simulink model "Clik_Jacobian_second_order"  (R2023a)
settings: Solver=VariableStepAuto  StartTime=0.0  StopTime=20  RelTol=1e-6
model workspace: external: MAT-File (data not in the file)
undefined symbols (not defined in the file): DiscIntNeverNeededParam, f_s
settings Model: Creator=benit  LastModifiedBy=Savio Del Peschio
settings OptimizationCC: ReuseModelBlockBuffer=off

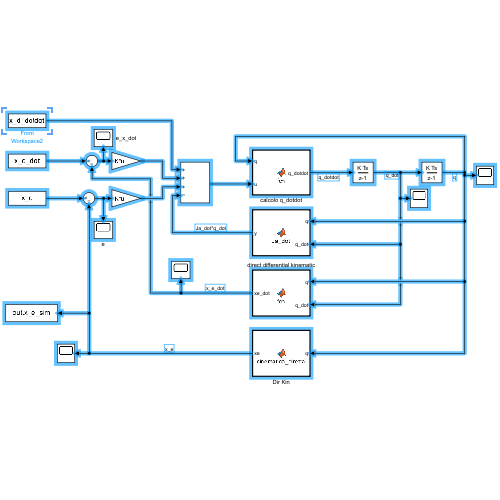
[thumbnail: Simulink's stored preview of the top-level diagram]
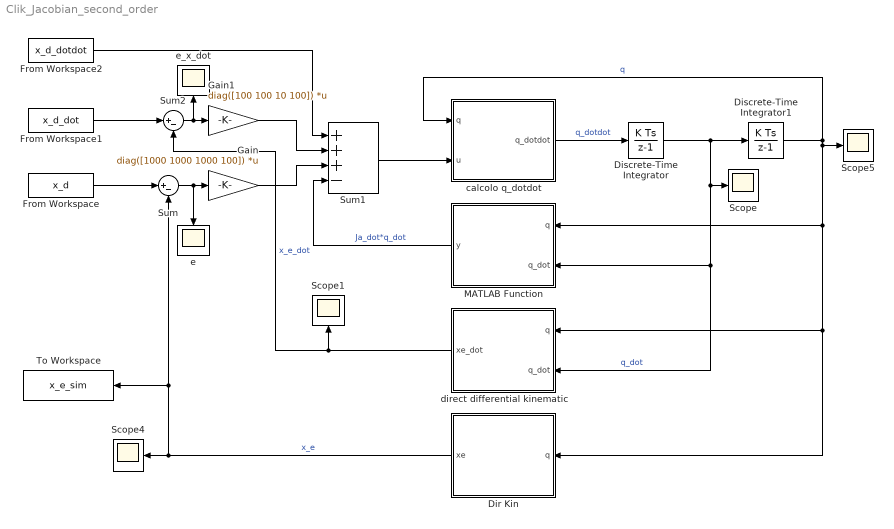
== system Clik_Jacobian_second_order ==
  Dir Kin : MATLAB Function  TreatAsAtomicUnit=on
  Discrete-Time Integrator : DiscreteIntegrator  gainval=1  InitialCondition=zeros(4,1)  SampleTime=1/f_s  ICPrevOutput=DiscIntNeverNeededParam  ICPrevScaledInput=DiscIntNeverNeededParam
  Discrete-Time Integrator1 : DiscreteIntegrator  gainval=1  InitialCondition=config_p_init'  SampleTime=1/f_s  ICPrevOutput=DiscIntNeverNeededParam  ICPrevScaledInput=DiscIntNeverNeededParam
  From Workspace : FromWorkspace  VariableName=x_d
  From Workspace1 : FromWorkspace  VariableName=x_d_dot
  From Workspace2 : FromWorkspace  VariableName=x_d_dotdot
  Gain : Gain  Gain=diag([1000 1000 1000 100])  Multiplication=Matrix(K*u)
  Gain1 : Gain  Gain=diag([100 100 10 100])  Multiplication=Matrix(K*u)
  MATLAB Function : MATLAB Function  TreatAsAtomicUnit=on
  Scope{,1,4..5} (4 alike) : Scope
  Sum : Sum  Inputs=|+-
  Sum1 : Sum  Inputs=+++-
  Sum2 : Sum  Inputs=|+-
  To Workspace : ToWorkspace  VariableName=x_e_sim  SaveFormat=Timeseries  SampleTime=-1
  calcolo q_dotdot : MATLAB Function  TreatAsAtomicUnit=on
  direct differential kinematic : MATLAB Function  TreatAsAtomicUnit=on
  e : Scope
  e_x_dot : Scope
  wires:
  calcolo q_dotdot/1(q_dotdot) -> Discrete-Time Integrator/1  "q_dotdot"
  From Workspace/1 -> Sum/1
  Dir Kin/1(xe) -> To Workspace/1, Sum/2, Scope4/1  "x_e"
  From Workspace1/1 -> Sum2/1
  Sum2/1 -> e_x_dot/1, Gain1/1
  From Workspace2/1 -> Sum1/1
  Gain1/1 -> Sum1/2
  Gain/1 -> Sum1/3
  direct differential kinematic/1(xe_dot) -> Sum2/2, Scope1/1  "x_e_dot"
  Sum1/1 -> calcolo q_dotdot/2(u)
  MATLAB Function/1(y) -> Sum1/4  "Ja_dot*q_dot"
  Discrete-Time Integrator/1 -> direct differential kinematic/2(q_dot), MATLAB Function/2(q_dot), Scope/1, Discrete-Time Integrator1/1  "q_dot"
  Discrete-Time Integrator1/1 -> Scope5/1, Dir Kin/1(q), direct differential kinematic/1(q), MATLAB Function/1(q), calcolo q_dotdot/1(q)  "q"
  Sum/1 -> e/1, Gain/1

== matlab function Clik_Jacobian_second_order/calcolo q_dotdot ==
  data: q input; u input; q_dotdot output
function q_dotdot = fcn(q,u)

    J = [-0.5*sin(q(1))-0.5*sin(q(1)+q(2))   -0.5*sin(q(1)+q(2))    0  0 
          0.5*cos(q(1))+0.5*cos(q(1)+q(2))    0.5*cos(q(1)+q(2))    0  0 
          0                                   0                    -1  0
          1                                   1                     0  -1];
    
    q_dotdot = pinv(J)*u;

end

== matlab function Clik_Jacobian_second_order/Dir Kin ==
  data: q input; xe output
function xe = cinematica_diretta(q)
    
    xe = [  0.5*cos(q(1))+0.5*cos(q(1)+q(2));
            0.5*sin(q(1))+0.5*sin(q(1)+q(2));
            1/2-q(3)
            q(1)+q(2)-q(4) ];

end

== matlab function Clik_Jacobian_second_order/direct differential kinematic ==
  data: q input; q_dot input; xe_dot output
function xe_dot = fcn(q,q_dot)

 Ja = [-0.5*sin(q(1))-0.5*sin(q(1)+q(2)) -0.5*sin(q(1)+q(2))    0 0
      0.5*cos(q(1))+0.5*cos(q(1)+q(2))  0.5*cos(q(1)+q(2))     0 0
      0                                0                    -1 0
      1                                1                    0 -1];

xe_dot = Ja*q_dot;

end

== matlab function Clik_Jacobian_second_order/MATLAB Function ==
  data: q input; q_dot input; y output
function y = Ja_dot(q, q_dot)

    J_min_dot = [-0.5*(q_dot(1)+q_dot(2))*cos(q(1)+q(2))-0.5*q_dot(1)*cos(q(1))              -0.5*(q_dot(1)+q_dot(2))*cos(q(1)+q(2))  0   0
                 -0.5*(q_dot(1)+q_dot(2))*sin(q(1)+q(2))-0.5*q_dot(1)*sin(q(1))              -0.5*(q_dot(1)+q_dot(2))*sin(q(1)+q(2))  0   0
                 0                                                                            0                                       0   0
                 0                                                                            0                                       0   0];
    
     y = J_min_dot*q_dot;
     
end
